simulink model "tunnel_diode"  (R2022b)
settings: Solver=VariableStepAuto  StartTime=0.0  StopTime=20  RelTol=1e-3
values from neighbouring files (symbols this model uses):
  A = [0  1/Cap ... (first row only)    [tunnel_diode_param.m]
  B = [0 ... (first row only)    [tunnel_diode_param.m]
  C = [1 0]    [tunnel_diode_param.m]
  F = [-1/Cap ... (first row only)    [tunnel_diode_param.m]
  x0 = [0; 0]    [tunnel_diode_param.m]
settings Model: Creator=alexe  LastModifiedBy=alexe

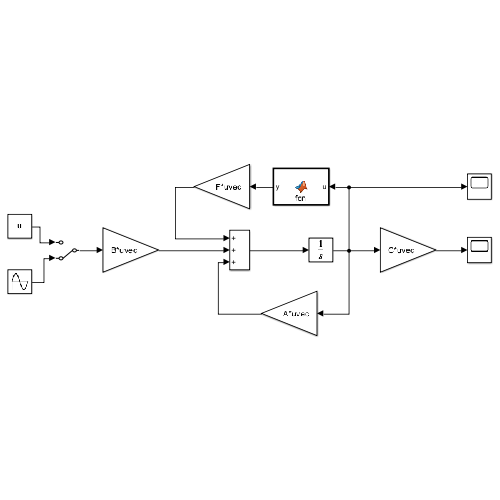
[thumbnail: Simulink's stored preview of the top-level diagram]
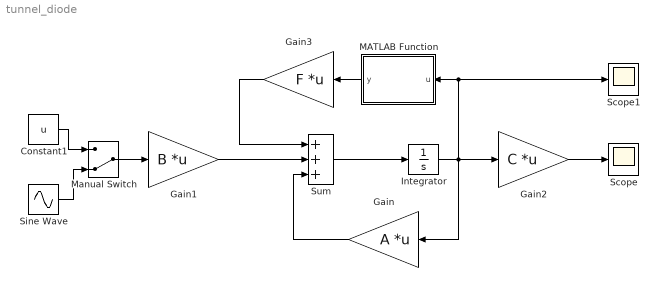
== system tunnel_diode ==
  Constant1 : Constant  Value=u
  Gain : Gain  Gain=A  Multiplication=Matrix(K*u) (u vector)
  Gain1 : Gain  Gain=B  Multiplication=Matrix(K*u) (u vector)
  Gain2 : Gain  Gain=C  Multiplication=Matrix(K*u) (u vector)
  Gain3 : Gain  Gain=F  Multiplication=Matrix(K*u) (u vector)
  Integrator : Integrator  InitialCondition=x0
  MATLAB Function : MATLAB Function  TreatAsAtomicUnit=on
  Manual Switch : ManualSwitch  CurrentSetting=0
  Scope : Scope
  Scope1 : Scope
  Sine Wave : Sin  Amplitude=u  SampleTime=0
  Sum : Sum  Inputs=+++
  wires:
  Integrator/1 -> MATLAB Function/1(u), Scope1/1, Gain/1, Gain2/1
  Sum/1 -> Integrator/1
  Gain1/1 -> Sum/2
  Gain/1 -> Sum/3
  MATLAB Function/1(y) -> Gain3/1
  Gain3/1 -> Sum/1
  Gain2/1 -> Scope/1
  Manual Switch/1 -> Gain1/1
  Constant1/1 -> Manual Switch/1
  Sine Wave/1 -> Manual Switch/2

== matlab function tunnel_diode/MATLAB Function ==
  data: u input; y output
function y = fcn(u)
x1 = u(1);
y = 17.76*x1 +-103.79*power(x1, 2) + 229.62*power(x1, 3) - 226.31*power(x1, 4) + 83.72*power(x1, 5);
